simulink model "ModelF_alt"  (R2018a)
settings: Solver=ode23tb  StartTime=0.0  StopTime=1  MaxStep=10e-6  RelTol=1e-3
values from neighbouring files (symbols this model uses):
  WidthP = 60    [parameter_set.m]
libraries: powerlib x20, simulink x1, powerlib_meascontrol x1
settings Model: Creator=Simon  LastModifiedBy=ivank
settings SolverCC: InitialStep=10e-8

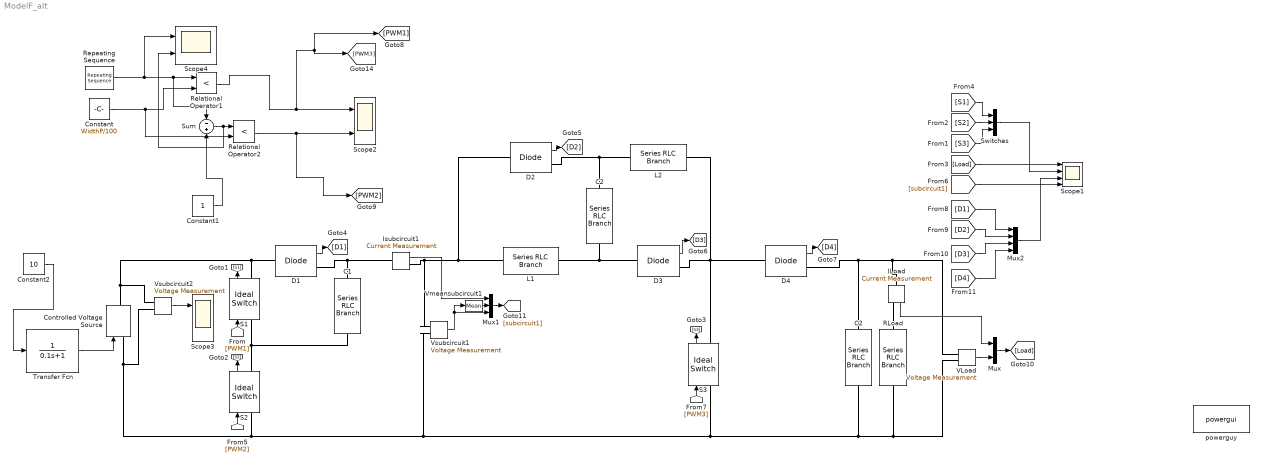
== system ModelF_alt ==
  C1 : powerlib/Elements/Series RLC Branch  LConnTagsString=__new0  RConnTagsString=__new0  BranchType=C  Resistance=1  Inductance=1e-3  SetiL0=off  InitialCurrent=0  Capacitance=220e-5  Setx0=off  InitialVoltage=0  Measurements=None
  C2 : powerlib/Elements/Series RLC Branch  LConnTagsString=__new0  RConnTagsString=__new0  BranchType=C  Resistance=1  Inductance=1e-3  SetiL0=off  InitialCurrent=0  Capacitance=220e-5  Setx0=off  InitialVoltage=0  Measurements=None
  "C2 " : powerlib/Elements/Series RLC Branch  LConnTagsString=__new0  RConnTagsString=__new0  BranchType=C  Resistance=1  Inductance=1e-3  SetiL0=off  InitialCurrent=0  Capacitance=220e-5  Setx0=off  InitialVoltage=0  Measurements=None
  Constant : Constant  Value=WidthP/100
  Constant1 : Constant
  Constant2 : Constant  Value=10
  Controlled Voltage Source : powerlib/Electrical Sources/Controlled Voltage Source  Initialize=on  Source_Type=AC  Amplitude=0  Phase=0  Frequency=0  Measurements=Voltage
  D{1..4} (4 alike) : powerlib/Power Electronics/Diode  Ron=0.001  Lon=0  Vf=0.8  IC=0  UseSnubber=0  Rs=500  Cs=250e-9  Measurements=on
  ILoad : powerlib/Measurements/Current Measurement  PhasorSimulation=off  OutputType=Complex  PSBequivalent=0
  Isubcircuit1 : powerlib/Measurements/Current Measurement  PhasorSimulation=off  OutputType=Complex  PSBequivalent=0
  L1 : powerlib/Elements/Series RLC Branch  LConnTagsString=__new0  RConnTagsString=__new0  BranchType=L  Resistance=1  Inductance=150e-6  SetiL0=off  InitialCurrent=0  Capacitance=1e-6  Setx0=off  InitialVoltage=0  Measurements=None
  L2 : powerlib/Elements/Series RLC Branch  LConnTagsString=__new0  RConnTagsString=__new0  BranchType=L  Resistance=1  Inductance=150e-6  SetiL0=off  InitialCurrent=0  Capacitance=1e-6  Setx0=off  InitialVoltage=0  Measurements=None
  Mux : Mux  Inputs=2
  Mux1 : Mux  Inputs=3
  Mux2 : Mux
  RLoad : powerlib/Elements/Series RLC Branch  LConnTagsString=__new0  RConnTagsString=__new0  BranchType=R  Resistance=225  Inductance=1e-3  SetiL0=off  InitialCurrent=0  Capacitance=1e-6  Setx0=off  InitialVoltage=0  Measurements=None
  Relational Operator1 : RelationalOperator  Operator=<  OutDataTypeStr=boolean  RndMeth=Simplest
  Relational Operator2 : RelationalOperator  Operator=<  OutDataTypeStr=boolean  RndMeth=Simplest
  Repeating Sequence : simulink/Sources/Repeating Sequence  rep_seq_t=[0 1/2 1]*(1/50000)  rep_seq_y=[0 1 0]
  S1 : powerlib/Power Electronics/Ideal Switch  Ron=0.00001  Lon=0  IC=0  Rs=1e9  Cs=inf  Measurements=on
  S2 : powerlib/Power Electronics/Ideal Switch  Ron=0.00001  Lon=0  IC=0  Rs=1e9  Cs=inf  Measurements=on
  S3 : powerlib/Power Electronics/Ideal Switch  Ron=0.00001  Lon=0  IC=0  Rs=1e9  Cs=inf  Measurements=on
  Scope1 : Scope  NumInputPorts=4
  Scope2 : Scope  NumInputPorts=2
  Scope3 : Scope  NumInputPorts=2
  Scope4 : Scope  NumInputPorts=2
  Sum : Sum  Inputs=-+
  Switches : Mux  Inputs=3
  Transfer Fcn : TransferFcn  Denominator=[0.1 1]
  VLoad : powerlib/Measurements/Voltage Measurement  PhasorSimulation=off  OutputType=Complex  PSBequivalent=0
  Vmeansubcircuit1 : powerlib_meascontrol/Measurements/Mean  Freq=1000  Vinit=0  Ts=0
  Vsubcircuit1 : powerlib/Measurements/Voltage Measurement  PhasorSimulation=off  OutputType=Complex  PSBequivalent=0
  Vsubcircuit2 : powerlib/Measurements/Voltage Measurement  PhasorSimulation=off  OutputType=Complex  PSBequivalent=0
  powerguy : powerlib/powergui  Priority=1  SimulationMode=Continuous  SampleTime=50e-6  frequency=60  Iterations=50  frequencyindice=0  Pbase=100e6  ErrMax=1e-4  UnitsV=kV  UnitsW=MW  buscounter=0  FunctionMessages=off  echomessages=off  EnableUseOfTLC=off  CurrentSourceSwitches=off  DisableSnubberDevices=off  DisableRonSwitches=off  DisableVfSwitches=off  DisplayEquations=off  SolverType=Tustin/Backward Euler (TBE)  Interpol=off  ExternalGateDelay=off  methode=off  Ts=100  x0status=blocks  SPID=on  SwTol=0  HookPort=off  RestoreLinks=warning  ResistiveCurrentMeasurement=off  Frange=[0:2:500]  Ylog=off  Xlog=on  ShowGrid=off  save=off  variable=ZData  structure=0  ZoomFFT=off  StartTime=0.0  cycles=1  DisplayStyle=1  fundamental=60  FreqAxis=off  MaxFrequency=1000  frequencyindicesteady=1  RmsSteady=1  display=off
  wires:
  Mux/1 -> [Load]
  ILoad/1 -> Mux/1
  VLoad/1 -> Mux/2
  S1/1 -> [S1]
  S2/1 -> [S2]
  S3/1 -> [S3]
  D1/1 -> [D1]
  D2/1 -> [D2]
  D3/1 -> [D3]
  D4/1 -> [D4]
  [S1] -> Switches/1
  [S2] -> Switches/2
  [S3] -> Switches/3
  Switches/1 -> Scope1/2
  [PWM1] -> S1/1
  [PWM2] -> S2/1
  Mux1/1 -> [subcircuit1]
  Isubcircuit1/1 -> Mux1/1
  Vsubcircuit1/1 -> Vmeansubcircuit1/1, Mux1/3
  Relational Operator2/1 -> [PWM2], Scope2/2
  [subcircuit1] -> Scope1/4
  Vmeansubcircuit1/1 -> Mux1/2
  [Load] -> Scope1/1
  Constant/1 -> Relational Operator2/2, Relational Operator1/2
  Sum/1 -> Scope4/2, Relational Operator2/1
  Repeating Sequence/1 -> Scope4/1, Sum/1, Relational Operator1/1
  Constant1/1 -> Sum/2
  Relational Operator1/1 -> [PWM3], [PWM1], Scope2/1
  [PWM3] -> S3/1
  [D1] -> Mux2/1
  Mux2/1 -> Scope1/3
  [D2] -> Mux2/2
  [D4] -> Mux2/4
  [D3] -> Mux2/3
  Constant2/1 -> Transfer Fcn/1
  Transfer Fcn/1 -> Controlled Voltage Source/1
  Vsubcircuit2/1 -> Scope3/1
  connections:
  D1/LConn1 -- Vsubcircuit2/LConn1 -- Controlled Voltage Source/RConn1 -- S1/RConn1
  S1/LConn1 -- S2/RConn1 -- C1/RConn1
  L1/RConn1 -- D3/LConn1 -- C2/RConn1
  S2/LConn1 -- Vsubcircuit2/LConn2 -- Controlled Voltage Source/LConn1 -- Vsubcircuit1/LConn2 -- "C2 "/RConn1 -- VLoad/LConn2 -- RLoad/RConn1 -- S3/LConn1
  VLoad/LConn1 -- "C2 "/LConn1 -- D4/RConn1 -- ILoad/LConn1
  D1/RConn1 -- Isubcircuit1/LConn1 -- C1/LConn1
  C2/LConn1 -- L2/LConn1 -- D2/RConn1
  RLoad/LConn1 -- ILoad/RConn1
  D3/RConn1 -- D4/LConn1 -- L2/RConn1 -- S3/RConn1
  D2/LConn1 -- Isubcircuit1/RConn1 -- Vsubcircuit1/LConn1 -- L1/LConn1
